simulink model "quad2ACDCfull120"  (R2021a)
settings: Solver=VariableStepAuto  StartTime=0.0  StopTime=0.06  RelTol=1e-3
libraries: spsThyristorLib x4, spsVoltageMeasurementLib x2, spsACVoltageSourceLib x1, spsMeanLib x1, spsSeriesRLCLoadLib x1, spspowerguiLib x1
settings Model: Creator=user  LastModifiedBy=user

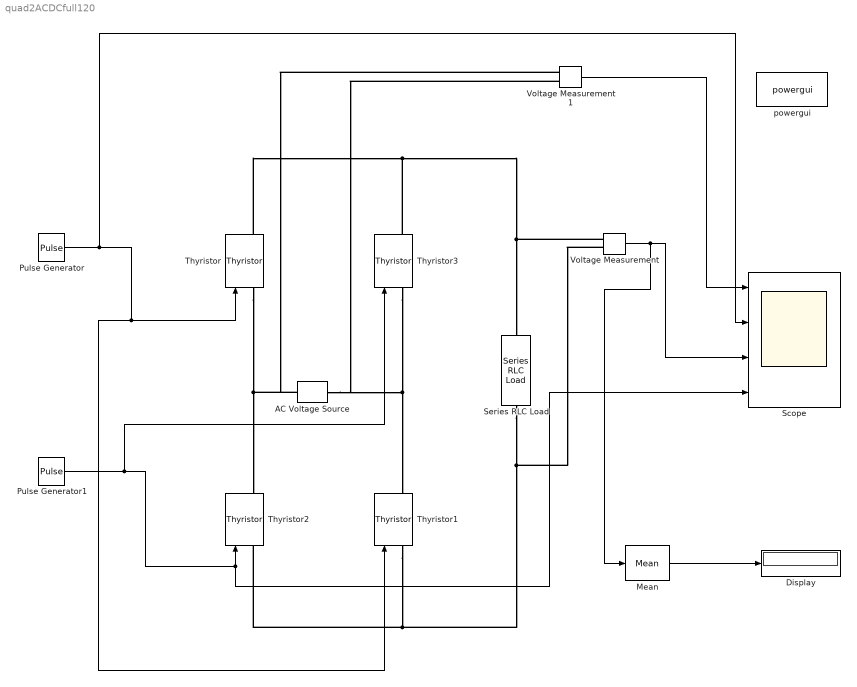
== system quad2ACDCfull120 ==
  AC Voltage Source : spsACVoltageSourceLib/AC Voltage Source  Amplitude=230*1.414  Phase=0  Frequency=50  SampleTime=0  Measurements=None  BusType=swing  Pref=10e3  Qref=0  Qmin=-inf  Qmax=+inf
  Display : Display
  Mean : spsMeanLib/Mean  Freq=60  Vinit=0  Ts=0
  Pulse Generator : DiscretePulseGenerator  PulseType=Time based  Amplitude=5  Period=20e-3  PulseWidth=10  PhaseDelay=6.666e-3
  Pulse Generator1 : DiscretePulseGenerator  PulseType=Time based  Amplitude=5  Period=20e-3  PulseWidth=10  PhaseDelay=16.666e-3
  Scope : Scope  NumInputPorts=4
  Series RLC Load : spsSeriesRLCLoadLib/Series RLC Load  LConnTagsString=a  RConnTagsString=__new0  NominalVoltage=230*1.414  NominalFrequency=50  ActivePower=500  InductivePower=666.6667  CapacitivePower=0  Setx0=off  InitialVoltage=0  SetiL0=off  InitialCurrent=0  Measurements=None  LoadType=constant Z
  Thyristor{,1..3} (4 alike) : spsThyristorLib/Thyristor  Ron=0.001  Lon=0  Vf=0.8  IC=0  Rs=500  Cs=250e-9  Measurements=on
  Voltage Measurement : spsVoltageMeasurementLib/Voltage Measurement  PhasorSimulation=off  OutputType=Complex  PSBequivalent=0
  Voltage Measurement1 : spsVoltageMeasurementLib/Voltage Measurement  PhasorSimulation=off  OutputType=Complex  PSBequivalent=0
  powergui : spspowerguiLib/powergui  Priority=1  SimulationMode=Continuous  SampleTime=50e-6  frequency=60  Iterations=50  frequencyindice=50  Pbase=100e6  ErrMax=1e-4  UnitsV=kV  UnitsW=MW  buscounter=0  FunctionMessages=off  echomessages=off  EnableUseOfTLC=off  CurrentSourceSwitches=off  DisableSnubberDevices=off  DisableRonSwitches=off  DisableVfSwitches=off  DisplayEquations=off  AutomaticDiscreteSolvers=off  SolverType=Tustin/Backward Euler (TBE)  Interpol=off  ExternalGateDelay=off  methode=off  Ts=100  x0status=blocks  SPID=on  SwTol=0  HookPort=off  NonlinearTolerance=1e-4  nMaxIteration=100  ContinueOnMaxIteration=off  RestoreLinks=warning  ResistiveCurrentMeasurement=off  Frange=[0:2:500]  Ylog=off  Xlog=on  ShowGrid=off  save=off  variable=ZData  structure=0  ZoomFFT=off  StartTime=0.0  cycles=1  DisplayStyle=1  fundamental=60  FreqAxis=off  MaxFrequency=1000  frequencyindicesteady=1  RmsSteady=1  display=off
  wires:
  Pulse Generator1/1 -> Thyristor3/1, Scope/4, Thyristor2/1
  Pulse Generator/1 -> Scope/2, Thyristor/1, Thyristor1/1
  Voltage Measurement/1 -> Mean/1, Scope/3
  Voltage Measurement1/1 -> Scope/1
  Mean/1 -> Display/1
  connections:
  Series RLC Load/RConn1 -- Voltage Measurement/LConn2 -- Thyristor1/LConn1 -- Thyristor2/LConn1
  Thyristor/LConn1 -- Voltage Measurement1/LConn1 -- AC Voltage Source/RConn1 -- Thyristor2/RConn1
  Thyristor3/LConn1 -- Voltage Measurement1/LConn2 -- AC Voltage Source/LConn1 -- Thyristor1/RConn1
  Thyristor/RConn1 -- Thyristor3/RConn1 -- Voltage Measurement/LConn1 -- Series RLC Load/LConn1
